simulink model "trackdraw"  (R2017a)
settings: Solver=VariableStepAuto  StartTime=0.0  StopTime=inf  RelTol=1e-3
libraries: robotlib x8
settings Model: Creator=fulei  LastModifiedBy=fulei

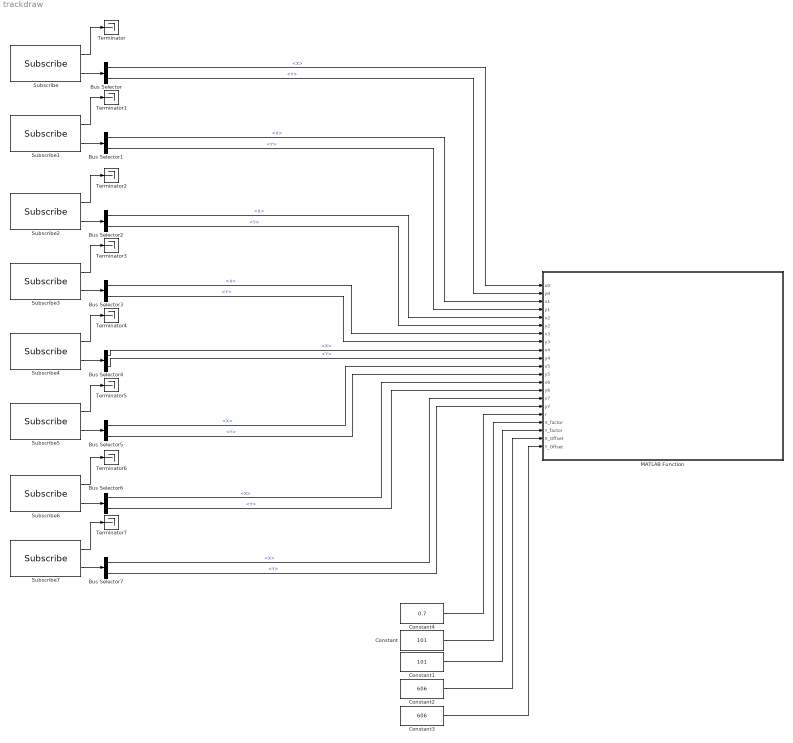
== system trackdraw ==
  Bus Selector{,1..7} (8 alike) : BusSelector  OutputSignals=Pose.Pose.Position.X,Pose.Pose.Position.Y
  Constant : Constant  Value=101
  Constant1 : Constant  Value=101
  Constant2 : Constant  Value=606
  Constant3 : Constant  Value=606
  Constant4 : Constant  Value=0.7
  MATLAB Function : MATLAB Function  TreatAsAtomicUnit=on
  Subscribe : robotlib/Subscribe  SourceLibraryInfo=This block requires Robotics System Toolbox  topicSource=Select from ROS network  topic=/robot_0/base_pose_ground_truth  messageType=nav_msgs/Odometry  sampleTime=-1  messageQueueLength=1
      settings: SourceProductBaseCode=RO
  Subscribe1 : robotlib/Subscribe  SourceLibraryInfo=This block requires Robotics System Toolbox  topicSource=Select from ROS network  topic=/robot_1/base_pose_ground_truth  messageType=nav_msgs/Odometry  sampleTime=-1  messageQueueLength=1
      settings: SourceProductBaseCode=RO
  Subscribe2 : robotlib/Subscribe  SourceLibraryInfo=This block requires Robotics System Toolbox  topicSource=Select from ROS network  topic=/robot_2/base_pose_ground_truth  messageType=nav_msgs/Odometry  sampleTime=-1  messageQueueLength=1
      settings: SourceProductBaseCode=RO
  Subscribe3 : robotlib/Subscribe  SourceLibraryInfo=This block requires Robotics System Toolbox  topicSource=Select from ROS network  topic=/robot_3/base_pose_ground_truth  messageType=nav_msgs/Odometry  sampleTime=-1  messageQueueLength=1
      settings: SourceProductBaseCode=RO
  Subscribe4 : robotlib/Subscribe  SourceLibraryInfo=This block requires Robotics System Toolbox  topicSource=Select from ROS network  topic=/robot_4/base_pose_ground_truth  messageType=nav_msgs/Odometry  sampleTime=-1  messageQueueLength=1
      settings: SourceProductBaseCode=RO
  Subscribe5 : robotlib/Subscribe  SourceLibraryInfo=This block requires Robotics System Toolbox  topicSource=Select from ROS network  topic=/robot_5/base_pose_ground_truth  messageType=nav_msgs/Odometry  sampleTime=-1  messageQueueLength=1
      settings: SourceProductBaseCode=RO
  Subscribe6 : robotlib/Subscribe  SourceLibraryInfo=This block requires Robotics System Toolbox  topicSource=Select from ROS network  topic=/robot_6/base_pose_ground_truth  messageType=nav_msgs/Odometry  sampleTime=-1  messageQueueLength=1
      settings: SourceProductBaseCode=RO
  Subscribe7 : robotlib/Subscribe  SourceLibraryInfo=This block requires Robotics System Toolbox  topicSource=Select from ROS network  topic=/robot_7/base_pose_ground_truth  messageType=nav_msgs/Odometry  sampleTime=-1  messageQueueLength=1
      settings: SourceProductBaseCode=RO
  Terminator{,1..7} (8 alike) : Terminator
  wires:
  Constant/1 -> MATLAB Function/18(X_factor)
  Constant1/1 -> MATLAB Function/19(Y_factor)
  Constant2/1 -> MATLAB Function/20(X_Offset)
  Constant3/1 -> MATLAB Function/21(Y_Offset)
  Subscribe/1 -> Terminator/1
  Subscribe/2 -> Bus Selector/1
  Bus Selector/1 -> MATLAB Function/1(x0)  "<X>"
  Bus Selector/2 -> MATLAB Function/2(y0)  "<Y>"
  Constant4/1 -> MATLAB Function/17(r)
  Subscribe1/2 -> Bus Selector1/1
  Subscribe1/1 -> Terminator1/1
  Bus Selector1/1 -> MATLAB Function/3(x1)  "<X>"
  Bus Selector1/2 -> MATLAB Function/4(y1)  "<Y>"
  Subscribe2/1 -> Terminator2/1
  Subscribe2/2 -> Bus Selector2/1
  Bus Selector2/1 -> MATLAB Function/5(x2)  "<X>"
  Bus Selector2/2 -> MATLAB Function/6(y2)  "<Y>"
  Bus Selector3/1 -> MATLAB Function/7(x3)  "<X>"
  Bus Selector3/2 -> MATLAB Function/8(y3)  "<Y>"
  Subscribe3/1 -> Terminator3/1
  Subscribe3/2 -> Bus Selector3/1
  Bus Selector4/1 -> MATLAB Function/9(x4)  "<X>"
  Bus Selector4/2 -> MATLAB Function/10(y4)  "<Y>"
  Subscribe4/1 -> Terminator4/1
  Subscribe4/2 -> Bus Selector4/1
  Bus Selector5/1 -> MATLAB Function/11(x5)  "<X>"
  Bus Selector5/2 -> MATLAB Function/12(y5)  "<Y>"
  Subscribe5/1 -> Terminator5/1
  Subscribe5/2 -> Bus Selector5/1
  Bus Selector6/1 -> MATLAB Function/13(x6)  "<X>"
  Bus Selector6/2 -> MATLAB Function/14(y6)  "<Y>"
  Subscribe6/1 -> Terminator6/1
  Subscribe6/2 -> Bus Selector6/1
  Bus Selector7/1 -> MATLAB Function/15(x7)  "<X>"
  Bus Selector7/2 -> MATLAB Function/16(y7)  "<Y>"
  Subscribe7/1 -> Terminator7/1
  Subscribe7/2 -> Bus Selector7/1

== matlab function trackdraw/MATLAB Function ==
  data: x0 input; y0 input; x1 input; y1 input; x2 input; y2 input; x3 input; y3 input; x4 input; y4 input; x5 input; y5 input; x6 input; y6 input; x7 input; y7 input; r input; X_factor input; Y_factor input; X_Offset input; Y_Offset input
function Gazebo_Track_Plotting(x0,y0,x1,y1,x2,y2,x3,y3,x4,y4,x5,y5,x6,y6,x7,y7,r,X_factor,Y_factor,X_Offset,Y_Offset)
hold on

%计算偏移量
rectangle('Position',[(-y0*X_factor+X_Offset)-r,(-x0*Y_factor+X_Offset)-r,2*r,2*r],'Curvature',[0,0],'LineWidth',3,'FaceColor','y','EdgeColor','r'),axis equal

rectangle('Position',[(-y1*X_factor+X_Offset)-r,(-x1*Y_factor+Y_Offset)-r,2*r,2*r],'Curvature',[0,0],'LineWidth',3,'FaceColor','y','EdgeColor','g'),axis equal

rectangle('Position',[(-y2*X_factor+X_Offset)-r,(-x2*Y_factor+X_Offset)-r,2*r,2*r],'Curvature',[1,1],'LineWidth',3,'LineStyle','--','FaceColor','y','EdgeColor','b'),axis equal

rectangle('Position',[(-y3*X_factor+X_Offset)-r,(-x3*Y_factor+Y_Offset)-r,2*r,2*r],'Curvature',[1,1],'LineWidth',3,'LineStyle','--','FaceColor','y','EdgeColor','c'),axis equal

rectangle('Position',[(-y4*X_factor+X_Offset)-r,(-x4*Y_factor+X_Offset)-r,2*r,2*r],'Curvature',[1,1],'LineWidth',3,'LineStyle','--','FaceColor','y','EdgeColor','m'),axis equal

rectangle('Position',[(-y5*X_factor+X_Offset)-r,(-x5*Y_factor+Y_Offset)-r,2*r,2*r],'Curvature',[0.5,1],'LineWidth',3,'LineStyle',':','FaceColor','y','EdgeColor','y'),axis equal

%rectangle('Position',[(-y6*X_factor+X_Offset)-r,(-x6*Y_factor+X_Offset)-r,2*r,2*r],'Curvature',[0.5,1],'LineWidth',3,'LineStyle',':','FaceColor','y','EdgeColor','k'),axis equal

%rectangle('Position',[(-y7*X_factor+X_Offset)-r,(-x7*Y_factor+Y_Offset)-r,2*r,2*r],'Curvature',[0.5,1],'LineWidth',3,'LineStyle',':','FaceColor','y','EdgeColor','w'),axis equal



end
